simulink model "Likitha_Version_8_1"  (R2025b)
settings: Solver=VariableStepAuto  StartTime=0.0  StopTime=0.3  RelTol=1e-3
undefined symbols (not defined in the file): Ion, Lithium
libraries: spsBatteryLib x50, spsSeriesRLCBranchLib x15, spsCurrentMeasurementLib x10, spsVoltageMeasurementLib x10, spsIdealSwitchLib x9, spsMosfetLib x7, slpidlib x4, spsPWMGeneratorDCDCLib x2, spspowerguiLib x2, spsACVoltageSourceLib x1, eeHysteresisControl x1, spsDCMachineLib x1
(part 3 of 4)

== system Likitha_Version_8_1/Subsystem11/4 ==
  Battery1 : spsBatteryLib/Battery  BatType=Lithium-Ion  NomV=3.3  NomQ=2.7  SOC=98.5  Batt_Tr=30  PresetModel=on  MaxQ=2.7  MinV=2.475  FullV=3.8412  Dis_rate=1.1739  R=0.012222  Normal_OP=2.4417  expZone="[3.5653     0.13265]"
  Bus Selector : BusSelector  OutputSignals=SOC (%),Current (A),Voltage (V)
  Product : Product
  Scope : Scope  NumInputPorts=4
      settings: ActiveDisplayYMinimum=99.92989  ActiveDisplayYMaximum=100.00779
  + : PMIOPort  Side=Right
  - : PMIOPort  Port=2  Side=Right
  tag scope: cm_4=global, soc4=global, vm_4=global
  wires:
  Battery1/1 -> Bus Selector/1
  Bus Selector/1 -> [soc4], Scope/1  "<SOC (%)>"
  Product/1 -> Scope/4
  Bus Selector/2 -> [cm_4], Product/1, Scope/2  "<Current (A)>"
  Bus Selector/3 -> [vm_4], Scope/3, Product/2  "<Voltage (V)>"
  connections:
  +/RConn1 -- Battery1/LConn1
  -/RConn1 -- Battery1/LConn2

== system Likitha_Version_8_1/Subsystem11/40 ==
  Battery1 : spsBatteryLib/Battery  BatType=Lithium-Ion  NomV=3.21  NomQ=2.52  SOC=72  Batt_Tr=30  PresetModel=on  MaxQ=2.52  MinV=2.4075  FullV=3.7364  Dis_rate=1.0957  R=0.012738  Normal_OP=2.279  expZone="[3.468     0.12381]"
  Bus Selector : BusSelector  OutputSignals=SOC (%),Current (A),Voltage (V)
  Product : Product
  Scope : Scope  NumInputPorts=4
      settings: ActiveDisplayYMinimum=99.92989  ActiveDisplayYMaximum=100.00779
  + : PMIOPort  Side=Right
  - : PMIOPort  Port=2  Side=Right
  tag scope: cm_29=global, soc29=global, vm_29=global
  wires:
  Battery1/1 -> Bus Selector/1
  Bus Selector/1 -> [soc29], Scope/1  "<SOC (%)>"
  Product/1 -> Scope/4
  Bus Selector/2 -> [cm_29], Product/1, Scope/2  "<Current (A)>"
  Bus Selector/3 -> [vm_29], Scope/3, Product/2  "<Voltage (V)>"
  connections:
  +/RConn1 -- Battery1/LConn1
  -/RConn1 -- Battery1/LConn2

== system Likitha_Version_8_1/Subsystem11/41 ==
  Battery1 : spsBatteryLib/Battery  BatType=Lithium-Ion  NomV=3.15  NomQ=2.4  SOC=65  Batt_Tr=30  PresetModel=on  MaxQ=2.4  MinV=2.3625  FullV=3.6666  Dis_rate=1.0435  R=0.013125  Normal_OP=2.1704  expZone="[3.4032     0.11791]"
  Bus Selector : BusSelector  OutputSignals=SOC (%),Current (A),Voltage (V)
  Product : Product
  Scope : Scope  NumInputPorts=4
      settings: ActiveDisplayYMinimum=99.92989  ActiveDisplayYMaximum=100.00779
  Series RLC Branch : spsSeriesRLCBranchLib/Series RLC Branch  LConnTagsString=__new0  RConnTagsString=__new0  BranchType=R  Resistance=0.01  Inductance=1e-3  SetiL0=off  InitialCurrent=0  Capacitance=1e-6  Setx0=off  InitialVoltage=0  Measurements=None
  + : PMIOPort  Side=Right
  - : PMIOPort  Port=2  Side=Right
  tag scope: cm_41=global, soc41=global, vm_41=global
  wires:
  Battery1/1 -> Bus Selector/1
  Bus Selector/1 -> [soc41], Scope/1  "<SOC (%)>"
  Product/1 -> Scope/4
  Bus Selector/2 -> [cm_41], Product/1, Scope/2  "<Current (A)>"
  Bus Selector/3 -> [vm_41], Scope/3, Product/2  "<Voltage (V)>"
  connections:
  -/RConn1 -- Battery1/LConn2
  Series RLC Branch/LConn1 -- Battery1/LConn1
  Series RLC Branch/RConn1 -- +/RConn1

== system Likitha_Version_8_1/Subsystem11/42 ==
  Battery1 : spsBatteryLib/Battery  BatType=Lithium-Ion  NomV=3.105  NomQ=2.31  SOC=56  Batt_Tr=30  PresetModel=on  MaxQ=2.31  MinV=2.3287  FullV=3.6142  Dis_rate=1.0043  R=0.013442  Normal_OP=2.089  expZone="[3.3546     0.11349]"
  Bus Selector : BusSelector  OutputSignals=SOC (%),Current (A),Voltage (V)
  Product : Product
  Scope : Scope  NumInputPorts=4
      settings: ActiveDisplayYMinimum=-1  ActiveDisplayYMaximum=1
  + : PMIOPort  Side=Right
  - : PMIOPort  Port=2  Side=Right
  tag scope: cm_50=global, soc50=global, vm_50=global
  wires:
  Battery1/1 -> Bus Selector/1
  Bus Selector/1 -> [soc50], Scope/1  "<SOC (%)>"
  Product/1 -> Scope/4
  Bus Selector/2 -> [cm_50], Product/1, Scope/2  "<Current (A)>"
  Bus Selector/3 -> [vm_50], Scope/3, Product/2  "<Voltage (V)>"
  connections:
  +/RConn1 -- Battery1/LConn1
  -/RConn1 -- Battery1/LConn2

== system Likitha_Version_8_1/Subsystem11/43 ==
  Battery1 : spsBatteryLib/Battery  BatType=Lithium-Ion  NomV=3.145  NomQ=2.39  SOC=64  Batt_Tr=30  PresetModel=on  MaxQ=2.39  MinV=2.3588  FullV=3.6607  Dis_rate=1.0391  R=0.013159  Normal_OP=2.1614  expZone="[3.3978     0.11742]"
  Bus Selector : BusSelector  OutputSignals=SOC (%),Current (A),Voltage (V)
  Product : Product
  Scope : Scope  NumInputPorts=4
      settings: ActiveDisplayYMinimum=99.92989  ActiveDisplayYMaximum=100.00779
  + : PMIOPort  Side=Right
  - : PMIOPort  Port=2  Side=Right
  tag scope: cm_42=global, soc42=global, vm_42=global
  wires:
  Battery1/1 -> Bus Selector/1
  Bus Selector/1 -> [soc42], Scope/1  "<SOC (%)>"
  Product/1 -> Scope/4
  Bus Selector/2 -> [cm_42], Product/1, Scope/2  "<Current (A)>"
  Bus Selector/3 -> [vm_42], Scope/3, Product/2  "<Voltage (V)>"
  connections:
  +/RConn1 -- Battery1/LConn1
  -/RConn1 -- Battery1/LConn2

== system Likitha_Version_8_1/Subsystem11/44 ==
  Battery1 : spsBatteryLib/Battery  BatType=Lithium-Ion  NomV=3.14  NomQ=2.38  SOC=63  Batt_Tr=30  PresetModel=on  MaxQ=2.38  MinV=2.355  FullV=3.6549  Dis_rate=1.0348  R=0.013193  Normal_OP=2.1523  expZone="[3.3924     0.11693]"
  Bus Selector : BusSelector  OutputSignals=SOC (%),Current (A),Voltage (V)
  Product : Product
  Scope : Scope  NumInputPorts=4
      settings: ActiveDisplayYMinimum=99.92989  ActiveDisplayYMaximum=100.00779
  + : PMIOPort  Side=Right
  - : PMIOPort  Port=2  Side=Right
  tag scope: cm_43=global, soc43=global, vm_43=global
  wires:
  Battery1/1 -> Bus Selector/1
  Bus Selector/1 -> [soc43], Scope/1  "<SOC (%)>"
  Product/1 -> Scope/4
  Bus Selector/2 -> [cm_43], Product/1, Scope/2  "<Current (A)>"
  Bus Selector/3 -> [vm_43], Scope/3, Product/2  "<Voltage (V)>"
  connections:
  +/RConn1 -- Battery1/LConn1
  -/RConn1 -- Battery1/LConn2

== system Likitha_Version_8_1/Subsystem11/45 ==
  Battery1 : spsBatteryLib/Battery  BatType=Lithium-Ion  NomV=3.135  NomQ=2.37  SOC=62  Batt_Tr=30  PresetModel=on  MaxQ=2.37  MinV=2.3512  FullV=3.6491  Dis_rate=1.0304  R=0.013228  Normal_OP=2.1433  expZone="[3.387     0.11644]"
  Bus Selector : BusSelector  OutputSignals=SOC (%),Current (A),Voltage (V)
  Product : Product
  Scope : Scope  NumInputPorts=4
      settings: ActiveDisplayYMinimum=99.92989  ActiveDisplayYMaximum=100.00779
  + : PMIOPort  Side=Right
  - : PMIOPort  Port=2  Side=Right
  tag scope: cm_44=global, soc44=global, vm_44=global
  wires:
  Battery1/1 -> Bus Selector/1
  Bus Selector/1 -> [soc44], Scope/1  "<SOC (%)>"
  Product/1 -> Scope/4
  Bus Selector/2 -> [cm_44], Product/1, Scope/2  "<Current (A)>"
  Bus Selector/3 -> [vm_44], Scope/3, Product/2  "<Voltage (V)>"
  connections:
  +/RConn1 -- Battery1/LConn1
  -/RConn1 -- Battery1/LConn2

== system Likitha_Version_8_1/Subsystem11/46 ==
  Battery1 : spsBatteryLib/Battery  BatType=Lithium-Ion  NomV=3.13  NomQ=2.36  SOC=61  Batt_Tr=30  PresetModel=on  MaxQ=2.36  MinV=2.3475  FullV=3.6433  Dis_rate=1.0261  R=0.013263  Normal_OP=2.1343  expZone="[3.3816     0.11595]"
  Bus Selector : BusSelector  OutputSignals=SOC (%),Current (A),Voltage (V)
  Product : Product
  Scope : Scope  NumInputPorts=4
      settings: ActiveDisplayYMinimum=99.92989  ActiveDisplayYMaximum=100.00779
  + : PMIOPort  Side=Right
  - : PMIOPort  Port=2  Side=Right
  tag scope: cm_45=global, soc45=global, vm_45=global
  wires:
  Battery1/1 -> Bus Selector/1
  Bus Selector/1 -> [soc45], Scope/1  "<SOC (%)>"
  Product/1 -> Scope/4
  Bus Selector/2 -> [cm_45], Product/1, Scope/2  "<Current (A)>"
  Bus Selector/3 -> [vm_45], Scope/3, Product/2  "<Voltage (V)>"
  connections:
  +/RConn1 -- Battery1/LConn1
  -/RConn1 -- Battery1/LConn2

== system Likitha_Version_8_1/Subsystem11/47 ==
  Battery1 : spsBatteryLib/Battery  BatType=Lithium-Ion  NomV=3.125  NomQ=2.35  SOC=60  Batt_Tr=30  PresetModel=on  MaxQ=2.35  MinV=2.3438  FullV=3.6375  Dis_rate=1.0217  R=0.013298  Normal_OP=2.1252  expZone="[3.3762     0.11546]"
  Bus Selector : BusSelector  OutputSignals=SOC (%),Current (A),Voltage (V)
  Product : Product
  Scope : Scope  NumInputPorts=4
      settings: ActiveDisplayYMinimum=99.92989  ActiveDisplayYMaximum=100.00779
  + : PMIOPort  Side=Right
  - : PMIOPort  Port=2  Side=Right
  tag scope: cm_46=global, soc46=global, vm_46=global
  wires:
  Battery1/1 -> Bus Selector/1
  Bus Selector/1 -> [soc46], Scope/1  "<SOC (%)>"
  Product/1 -> Scope/4
  Bus Selector/2 -> [cm_46], Product/1, Scope/2  "<Current (A)>"
  Bus Selector/3 -> [vm_46], Scope/3, Product/2  "<Voltage (V)>"
  connections:
  +/RConn1 -- Battery1/LConn1
  -/RConn1 -- Battery1/LConn2

== system Likitha_Version_8_1/Subsystem11/48 ==
  Battery1 : spsBatteryLib/Battery  BatType=Lithium-Ion  NomV=3.12  NomQ=2.34  SOC=59  Batt_Tr=30  PresetModel=on  MaxQ=2.34  MinV=2.34  FullV=3.6316  Dis_rate=1.0174  R=0.013333  Normal_OP=2.1162  expZone="[3.3708     0.11497]"
  Bus Selector : BusSelector  OutputSignals=SOC (%),Current (A),Voltage (V)
  Product : Product
  Scope : Scope  NumInputPorts=4
      settings: ActiveDisplayYMinimum=99.92989  ActiveDisplayYMaximum=100.00779
  + : PMIOPort  Side=Right
  - : PMIOPort  Port=2  Side=Right
  tag scope: cm_47=global, soc47=global, vm_47=global
  wires:
  Battery1/1 -> Bus Selector/1
  Bus Selector/1 -> [soc47], Scope/1  "<SOC (%)>"
  Product/1 -> Scope/4
  Bus Selector/2 -> [cm_47], Product/1, Scope/2  "<Current (A)>"
  Bus Selector/3 -> [vm_47], Scope/3, Product/2  "<Voltage (V)>"
  connections:
  +/RConn1 -- Battery1/LConn1
  -/RConn1 -- Battery1/LConn2

== system Likitha_Version_8_1/Subsystem11/49 ==
  Battery1 : spsBatteryLib/Battery  BatType=Lithium-Ion  NomV=3.115  NomQ=2.33  SOC=58  Batt_Tr=30  PresetModel=on  MaxQ=2.33  MinV=2.3363  FullV=3.6258  Dis_rate=1.013  R=0.013369  Normal_OP=2.1071  expZone="[3.3654     0.11447]"
  Bus Selector : BusSelector  OutputSignals=SOC (%),Current (A),Voltage (V)
  Product : Product
  Scope : Scope  NumInputPorts=4
      settings: ActiveDisplayYMinimum=99.92989  ActiveDisplayYMaximum=100.00779
  + : PMIOPort  Side=Right
  - : PMIOPort  Port=2  Side=Right
  tag scope: cm_48=global, soc48=global, vm_48=global
  wires:
  Battery1/1 -> Bus Selector/1
  Bus Selector/1 -> [soc48], Scope/1  "<SOC (%)>"
  Product/1 -> Scope/4
  Bus Selector/2 -> [cm_48], Product/1, Scope/2  "<Current (A)>"
  Bus Selector/3 -> [vm_48], Scope/3, Product/2  "<Voltage (V)>"
  connections:
  +/RConn1 -- Battery1/LConn1
  -/RConn1 -- Battery1/LConn2

== system Likitha_Version_8_1/Subsystem11/5 ==
  Battery1 : spsBatteryLib/Battery  BatType=Lithium-Ion  NomV=3.3  NomQ=2.7  SOC=98  Batt_Tr=30  PresetModel=on  MaxQ=2.7  MinV=2.475  FullV=3.8412  Dis_rate=1.1739  R=0.012222  Normal_OP=2.4417  expZone="[3.5653     0.13265]"
  Bus Selector : BusSelector  OutputSignals=SOC (%),Current (A),Voltage (V)
  Product : Product
  Scope : Scope  NumInputPorts=4
      settings: ActiveDisplayYMinimum=99.92989  ActiveDisplayYMaximum=100.00779
  + : PMIOPort  Side=Right
  - : PMIOPort  Port=2  Side=Right
  tag scope: cm_5=global, soc5=global, vm_5=global
  wires:
  Battery1/1 -> Bus Selector/1
  Bus Selector/1 -> [soc5], Scope/1  "<SOC (%)>"
  Bus Selector/2 -> Product/1, Scope/2  "<Current (A)>"
  Product/1 -> Scope/4
  Bus Selector/3 -> [vm_5], [cm_5], Scope/3, Product/2  "<Voltage (V)>"
  connections:
  +/RConn1 -- Battery1/LConn1
  -/RConn1 -- Battery1/LConn2

== system Likitha_Version_8_1/Subsystem11/50 ==
  Battery1 : spsBatteryLib/Battery  BatType=Lithium-Ion  NomV=3.11  NomQ=2.32  SOC=57  Batt_Tr=30  PresetModel=on  MaxQ=2.32  MinV=2.3325  FullV=3.62  Dis_rate=1.0087  R=0.013405  Normal_OP=2.0981  expZone="[3.36     0.11398]"
  Bus Selector : BusSelector  OutputSignals=SOC (%),Current (A),Voltage (V)
  Product : Product
  Scope : Scope  NumInputPorts=4
      settings: ActiveDisplayYMinimum=99.92989  ActiveDisplayYMaximum=100.00779
  + : PMIOPort  Side=Right
  - : PMIOPort  Port=2  Side=Right
  tag scope: cm_49=global, soc49=global, vm_49=global
  wires:
  Battery1/1 -> Bus Selector/1
  Bus Selector/1 -> [soc49], Scope/1  "<SOC (%)>"
  Product/1 -> Scope/4
  Bus Selector/2 -> [cm_49], Product/1, Scope/2  "<Current (A)>"
  Bus Selector/3 -> [vm_49], Scope/3, Product/2  "<Voltage (V)>"
  connections:
  +/RConn1 -- Battery1/LConn1
  -/RConn1 -- Battery1/LConn2

== system Likitha_Version_8_1/Subsystem11/6 ==
  Battery1 : spsBatteryLib/Battery  BatType=Lithium-Ion  NomV=3.3  NomQ=2.7  SOC=97.5  Batt_Tr=30  PresetModel=on  MaxQ=2.7  MinV=2.475  FullV=3.8412  Dis_rate=1.1739  R=0.012222  Normal_OP=2.4417  expZone="[3.5653     0.13265]"
  Bus Selector : BusSelector  OutputSignals=SOC (%),Current (A),Voltage (V)
  Product : Product
  Scope : Scope  NumInputPorts=4
      settings: ActiveDisplayYMinimum=99.92989  ActiveDisplayYMaximum=100.00779
  + : PMIOPort  Side=Right
  - : PMIOPort  Port=2  Side=Right
  tag scope: cm_6=global, soc6=global, vm_6=global
  wires:
  Battery1/1 -> Bus Selector/1
  Bus Selector/1 -> [soc6], Scope/1  "<SOC (%)>"
  Product/1 -> Scope/4
  Bus Selector/2 -> [cm_6], Product/1, Scope/2  "<Current (A)>"
  Bus Selector/3 -> [vm_6], Scope/3, Product/2  "<Voltage (V)>"
  connections:
  +/RConn1 -- Battery1/LConn1
  -/RConn1 -- Battery1/LConn2

== system Likitha_Version_8_1/Subsystem11/7 ==
  Battery1 : spsBatteryLib/Battery  BatType=Lithium-Ion  NomV=3.3  NomQ=2.7  SOC=97  Batt_Tr=30  PresetModel=on  MaxQ=2.7  MinV=2.475  FullV=3.8412  Dis_rate=1.1739  R=0.012222  Normal_OP=2.4417  expZone="[3.5653     0.13265]"
  Bus Selector : BusSelector  OutputSignals=SOC (%),Current (A),Voltage (V)
  Product : Product
  Scope : Scope  NumInputPorts=4
      settings: ActiveDisplayYMinimum=99.92989  ActiveDisplayYMaximum=100.00779
  + : PMIOPort  Side=Right
  - : PMIOPort  Port=2  Side=Right
  tag scope: cm_7=global, soc7=global, vm_7=global
  wires:
  Battery1/1 -> Bus Selector/1
  Bus Selector/1 -> [soc7], Scope/1  "<SOC (%)>"
  Product/1 -> Scope/4
  Bus Selector/2 -> [cm_7], Product/1, Scope/2  "<Current (A)>"
  Bus Selector/3 -> [vm_7], Scope/3, Product/2  "<Voltage (V)>"
  connections:
  +/RConn1 -- Battery1/LConn1
  -/RConn1 -- Battery1/LConn2

== system Likitha_Version_8_1/Subsystem11/8 ==
  Battery1 : spsBatteryLib/Battery  BatType=Lithium-Ion  NomV=3.3  NomQ=2.7  SOC=96.5  Batt_Tr=30  PresetModel=on  MaxQ=2.7  MinV=2.475  FullV=3.8412  Dis_rate=1.1739  R=0.012222  Normal_OP=2.4417  expZone="[3.5653     0.13265]"
  Bus Selector : BusSelector  OutputSignals=SOC (%),Current (A),Voltage (V)
  Product : Product
  Scope : Scope  NumInputPorts=4
      settings: ActiveDisplayYMinimum=99.92989  ActiveDisplayYMaximum=100.00779
  + : PMIOPort  Side=Right
  - : PMIOPort  Port=2  Side=Right
  tag scope: cm_8=global, soc8=global, vm_8=global
  wires:
  Battery1/1 -> Bus Selector/1
  Bus Selector/1 -> [soc8], Scope/1  "<SOC (%)>"
  Product/1 -> Scope/4
  Bus Selector/2 -> [cm_8], Product/1, Scope/2  "<Current (A)>"
  Bus Selector/3 -> Scope/3, [vm_8], Product/2  "<Voltage (V)>"
  connections:
  +/RConn1 -- Battery1/LConn1
  -/RConn1 -- Battery1/LConn2

== system Likitha_Version_8_1/Subsystem11/9 ==
  Battery1 : spsBatteryLib/Battery  BatType=Lithium-Ion  NomV=3.3  NomQ=2.7  SOC=96  Batt_Tr=30  PresetModel=on  MaxQ=2.7  MinV=2.475  FullV=3.8412  Dis_rate=1.1739  R=0.012222  Normal_OP=2.4417  expZone="[3.5653     0.13265]"
  Bus Selector : BusSelector  OutputSignals=SOC (%),Current (A),Voltage (V)
  Product : Product
  Scope : Scope  NumInputPorts=4
      settings: ActiveDisplayYMinimum=99.92989  ActiveDisplayYMaximum=100.00779
  + : PMIOPort  Side=Right
  - : PMIOPort  Port=2  Side=Right
  tag scope: cm_9=global, soc9=global, vm_9=global
  wires:
  Battery1/1 -> Bus Selector/1
  Bus Selector/1 -> [soc9], Scope/1  "<SOC (%)>"
  Product/1 -> Scope/4
  Bus Selector/2 -> [cm_9], Product/1, Scope/2  "<Current (A)>"
  Bus Selector/3 -> [vm_9], Scope/3, Product/2  "<Voltage (V)>"
  connections:
  +/RConn1 -- Battery1/LConn1
  -/RConn1 -- Battery1/LConn2

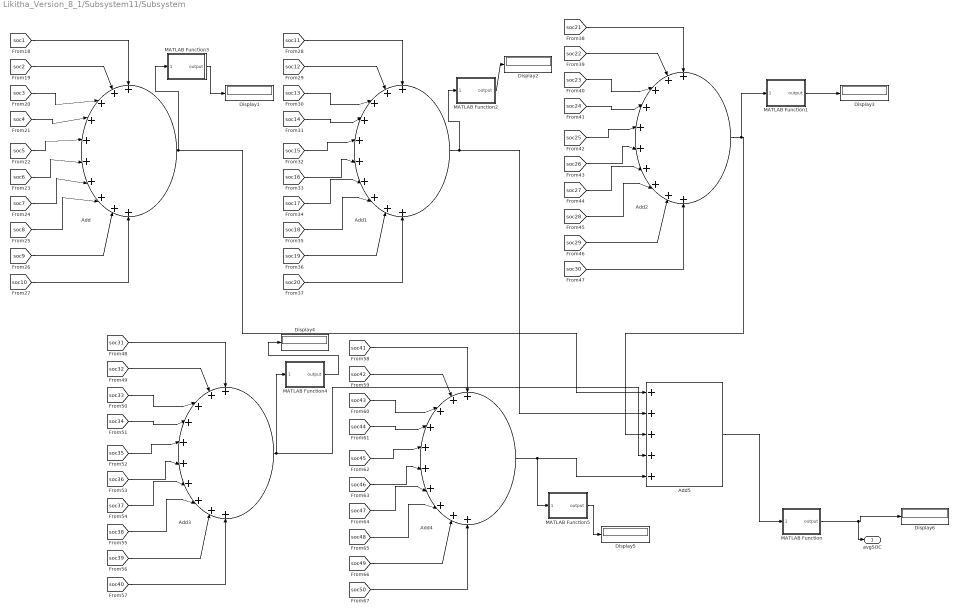
== system Likitha_Version_8_1/Subsystem11/Subsystem ==
  Add{,1..4} (5 alike) : Sum  Inputs=++++++++++
  Add5 : Sum  Inputs=+++++
  Display{1..6} (6 alike) : Display
  MATLAB Function : MATLAB Function  TreatAsAtomicUnit=on
  MATLAB Function1 : MATLAB Function  TreatAsAtomicUnit=on
  MATLAB Function2 : MATLAB Function  TreatAsAtomicUnit=on
  MATLAB Function3 : MATLAB Function  TreatAsAtomicUnit=on
  MATLAB Function4 : MATLAB Function  TreatAsAtomicUnit=on
  MATLAB Function5 : MATLAB Function  TreatAsAtomicUnit=on
  avgSOC : Outport
  wires:
  [soc16] -> Add1/6
  [soc31] -> Add3/1
  [soc42] -> Add4/2
  [soc6] -> Add/6
  Add3/1 -> MATLAB Function4/1(inputValue), Add5/4
  [soc33] -> Add3/3
  [soc12] -> Add1/2
  [soc50] -> Add4/10
  [soc1] -> Add/1
  [soc13] -> Add1/3
  [soc39] -> Add3/9
  Add2/1 -> MATLAB Function1/1(inputValue), Add5/3
  [soc28] -> Add2/8
  [soc3] -> Add/3
  [soc17] -> Add1/7
  [soc36] -> Add3/6
  [soc2] -> Add/2
  [soc45] -> Add4/5
  [soc49] -> Add4/9
  [soc27] -> Add2/7
  [soc48] -> Add4/8
  [soc15] -> Add1/5
  [soc20] -> Add1/10
  [soc43] -> Add4/3
  [soc26] -> Add2/6
  Add1/1 -> MATLAB Function2/1(inputValue), Add5/2
  [soc41] -> Add4/1
  [soc46] -> Add4/6
  [soc14] -> Add1/4
  [soc24] -> Add2/4
  [soc22] -> Add2/2
  [soc44] -> Add4/4
  [soc47] -> Add4/7
  [soc38] -> Add3/8
  [soc21] -> Add2/1
  [soc18] -> Add1/8
  [soc7] -> Add/7
  [soc19] -> Add1/9
  [soc9] -> Add/9
  [soc40] -> Add3/10
  [soc4] -> Add/4
  [soc11] -> Add1/1
  [soc35] -> Add3/5
  [soc8] -> Add/8
  Add/1 -> Add5/1, MATLAB Function3/1(inputValue)
  [soc5] -> Add/5
  [soc37] -> Add3/7
  [soc29] -> Add2/9
  Add4/1 -> MATLAB Function5/1(inputValue), Add5/5
  [soc34] -> Add3/4
  [soc32] -> Add3/2
  [soc10] -> Add/10
  [soc25] -> Add2/5
  [soc30] -> Add2/10
  [soc23] -> Add2/3
  Add5/1 -> MATLAB Function/1(inputValue)
  MATLAB Function/1(output) -> avgSOC/1, Display6/1
  MATLAB Function1/1(output) -> Display3/1
  MATLAB Function2/1(output) -> Display2/1
  MATLAB Function3/1(output) -> Display1/1
  MATLAB Function4/1(output) -> Display4/1
  MATLAB Function5/1(output) -> Display5/1

== system Likitha_Version_8_1/AC to DC/Subsystem1/Subsystem ==
  Iref : Inport
  Clock : Clock
  Constant : Constant  Value=2*pi/3
  Gain : Gain  Gain=2*pi*50
  Gain2 : Gain  Gain=2*pi*50
  Gain3 : Gain  Gain=2*pi*50
  Mux : Mux  Inputs=3
  Product : Product
  Sin : Trigonometry
  Sin1 : Trigonometry
  Sin2 : Trigonometry
  Subtract : Sum  Inputs=+-
  Subtract1 : Sum
  Out1 : Outport
  wires:
  Mux/1 -> Product/1
  Gain/1 -> Sin/1
  Sin2/1 -> Mux/3
  Clock/1 -> Gain3/1, Gain2/1, Gain/1
  Sin/1 -> Mux/1
  Constant/1 -> Subtract1/2, Subtract/2
  Subtract/1 -> Sin1/1
  Sin1/1 -> Mux/2
  Gain2/1 -> Subtract/1
  Gain3/1 -> Subtract1/1
  Subtract1/1 -> Sin2/1
  Product/1 -> Out1/1
  Iref/1 -> Product/2

== matlab function Likitha_Version_8_1/Subsystem11/MATLAB Function ==
  settings: updateMethod=DISCRETE
  data: V1 input; S1 output; V2 input; V3 input; V4 input; V5 input; S2 output; S3 output; S4 output; S5 output
function [S1,S2,S3,S4,S5] = battery_pack_switch_logic(V1,V2,V3,V4,V5)
% Outputs: 1 = ON, 0 = OFF

%% Parameters
V_over = 35;      % Over-voltage threshold
V_under = 30;     % Under-voltage threshold
V_tol = 0.5;      % Voltage balancing tolerance

V = [V1 V2 V3 V4 V5];

%% Persistent switch states (memory)
persistent S
if isempty(S)
    S = ones(1,5);   % All ON initially
end

%% Average voltage of active packs
V_active = V(S == 1);
if isempty(V_active)
    V_avg = mean(V);   % fallback
else
    V_avg = mean(V_active);
end

%% Control logic
for i = 1:5

    % Protection: Over / Under Voltage
    if V(i) > V_over || V(i) < V_under
        S(i) = 0;   % Force OFF
    end

    % Re-enable logic (balancing condition)
    if S(i) == 0
        if abs(V(i) - V_avg) <= V_tol
            S(i) = 1;   % Turn ON again
        end
    end

end

%% Outputs
S1 = S(1);
S2 = S(2);
S3 = S(3);
S4 = S(4);
S5 = S(5);

end

== matlab function Likitha_Version_8_1/Subsystem2/MATLAB Function1 ==
  settings: updateMethod=DISCRETE
  data: SOC input double size=1; windowData output double size=[100 22]; SOH input double size=1; SOP input double size=1; DOD input double size=1; ROH input double size=1; RUL input double size=1; CycleCount input double size=1; V_avg input double size=1; I_avg input double size=1; P_avg input double size=1; stress_idx input double size=1; aging_rate_frac input double size=1; energy_kWh input double size=1; degrad_idx input double size=1; T_idx input double size=1; health_idx input double size=1; I_peak input double size=1; V_min input double size=1; T_max input double size=1; Ah_charge_total input double size=1; Ah_discharge_total input double size=1; overtime_sec input double size=1; timestamp input double size=1; windowLabels output double size=[1 2]; dataValid output double size=1
function [windowData, windowLabels, dataValid] = PreTrainingData_Fixed(...
    SOC, SOH, SOP, DOD, ROH, RUL, CycleCount, ...
    V_avg, I_avg, P_avg, stress_idx, aging_rate_frac, energy_kWh, ...
    degrad_idx, T_idx, health_idx, I_peak, V_min, T_max, ...
    Ah_charge_total, Ah_discharge_total, overtime_sec, ...
    timestamp)

% Internal constants
windowSize = 100;   % number of samples per window
stepSize   = 0.1;   % time interval (s) between new windows

persistent buffer timeBuffer bufferIdx counter lastOutputTime
persistent firstRun

if isempty(firstRun)
    buffer = zeros(windowSize, 22);
    timeBuffer = zeros(windowSize, 1);
    bufferIdx = 1;
    counter = 0;
    lastOutputTime = -inf;
    firstRun = false;
end

% Current feature vector (1×22)
currentFeatures = [SOC, SOH, SOP, DOD, ROH, RUL, CycleCount, ...
                   V_avg, I_avg, P_avg, stress_idx, aging_rate_frac, energy_kWh, ...
                   degrad_idx, T_idx, health_idx, I_peak, V_min, T_max, ...
                   Ah_charge_total, Ah_discharge_total, overtime_sec];

% Store in circular buffer
buffer(bufferIdx, :) = currentFeatures;
timeBuffer(bufferIdx) = timestamp;
bufferIdx = mod(bufferIdx, windowSize) + 1;
counter = counter + 1;

% Default outputs (fixed size)
windowData = zeros(windowSize, 22);
windowLabels = [0, 0];
dataValid = 0;

% Check if we have a full window and enough time has passed
if counter >= windowSize && (timestamp - lastOutputTime) >= stepSize
    % Create index order for chronological order
    if bufferIdx > 1
        idxOrder = [bufferIdx:windowSize, 1:bufferIdx-1];
    else
        idxOrder = 1:windowSize;
    end
    % Fill windowData row by row (ensures fixed size)
    for i = 1:windowSize
        windowData(i, :) = buffer(idxOrder(i), :);
    end
    windowLabels = windowData(end, 1:2);
    dataValid = 1;
    lastOutputTime = timestamp;
end

end

== matlab function Likitha_Version_8_1/Subsystem2/MATLAB Function2 ==
  data: windowData input double size=[100 22]; SOC_pred output double size=1; windowLabels input double size=[1 2]; dataValid input double size=1; algorithmChoice input double size=1; SOH_pred output double size=1; RUL_pred output double size=1; confidence output double size=[1 2]; algoCode output double size=1; metrics output double size=[1 4]
function [SOC_pred, SOH_pred, RUL_pred, confidence, algoCode, metrics] = ...
    AI_ML_Estimator(windowData, windowLabels, dataValid, algorithmChoice)

% AI/ML/DL Estimator – fixed‑size, code‑generation compatible, no tic/toc
%
% Inputs:
%   windowData      : [100x22] matrix – most recent window of parameters
%   windowLabels    : [1x2] vector – [SOC, SOH] of the last sample in window
%   dataValid       : scalar – 1 when a new window is ready
%   algorithmChoice : scalar – 1=Linear, 2=Neural, 3=LSTM
%
% Outputs (all fixed size):
%   SOC_pred, SOH_pred, RUL_pred : scalars
%   confidence                    : [1x2] vector [conf_SOC, conf_SOH]
%   algoCode                      : scalar (0=None, 1=Linear, 2=Neural, 3=LSTM)
%   metrics                       : [1x4] vector [RMSE_SOC, RMSE_SOH, MAE_SOC, MAE_SOH]

% -------------------------------------------------------------------------
% Internal constants (must match Block 8)
windowSize = 100;
retrainInterval = 10;   % retrain every 'retrainInterval' new windows
% -------------------------------------------------------------------------

persistent X_buffer Y_buffer bufferIdx nSamples
persistent theta_SOC theta_SOH
persistent windowCount trainedAlgo

% Initialize all persistent variables
if isempty(X_buffer)
    X_buffer = zeros(windowSize, 22);
    Y_buffer = zeros(windowSize, 2);
    bufferIdx = 1;
    nSamples = 0;
    theta_SOC = zeros(22, 1);
    theta_SOH = zeros(22, 1);
    windowCount = 0;
    trainedAlgo = 0;
end

% Initialize outputs (to avoid "undefined on some paths")
SOC_pred = 0;
SOH_pred = 0;
RUL_pred = 0;
confidence = [0.5, 0.5];
algoCode = 0;
metrics = zeros(1, 4);   % ensures metrics is always defined

% If a new valid window arrives, store its last sample as a training point
if dataValid
    X_last = windowData(end, :);      % 1x22
    Y_last = windowLabels;             % 1x2

    % Store in circular buffer
    X_buffer(bufferIdx, :) = X_last;
    Y_buffer(bufferIdx, :) = Y_last;
    bufferIdx = mod(bufferIdx, windowSize) + 1;
    nSamples = min(nSamples + 1, windowSize);

    windowCount = windowCount + 1;
end

% Retrain when enough windows and sufficient samples
if dataValid && nSamples >= 30 && windowCount >= retrainInterval
    X_train = X_buffer(1:nSamples, :);
    Y_train = Y_buffer(1:nSamples, :);
    X_aug = [ones(nSamples, 1), X_train];   % add bias

    switch algorithmChoice
        case 1  % Linear Regression
            theta_SOC = (X_aug' * X_aug) \ (X_aug' * Y_train(:,1));
            theta_SOH = (X_aug' * X_aug) \ (X_aug' * Y_train(:,2));
            trainedAlgo = 1;

        case 2  % Neural Net (placeholder – use linear)
            theta_SOC = (X_aug' * X_aug) \ (X_aug' * Y_train(:,1));
            theta_SOH = (X_aug' * X_aug) \ (X_aug' * Y_train(:,2));
            trainedAlgo = 2;   % still linear for now

        case 3  % LSTM placeholder
            theta_SOC = (X_aug' * X_aug) \ (X_aug' * Y_train(:,1));
            theta_SOH = (X_aug' * X_aug) \ (X_aug' * Y_train(:,2));
            trainedAlgo = 3;
    end

    % Compute metrics
    Y_pred_SOC = X_aug * theta_SOC;
    Y_pred_SOH = X_aug * theta_SOH;
    rmse_soc = sqrt(mean((Y_train(:,1) - Y_pred_SOC).^2));
    rmse_soh = sqrt(mean((Y_train(:,2) - Y_pred_SOH).^2));
    mae_soc  = mean(abs(Y_train(:,1) - Y_pred_SOC));
    mae_soh  = mean(abs(Y_train(:,2) - Y_pred_SOH));
    metrics = [rmse_soc, rmse_soh, mae_soc, mae_soh];

    windowCount = 0;   % reset counter
end

% Make prediction using the most recent sample
X_pred = windowData(end, :);          % 1x22
X_pred_aug = [1, X_pred];             % add bias

if trainedAlgo >= 1
    SOC_pred = X_pred_aug * theta_SOC;
    SOH_pred = X_pred_aug * theta_SOH;
    confidence = [0.9, 0.9];
    algoCode = trainedAlgo;
else
    % No model yet – use the labels of the current window
    SOC_pred = windowLabels(1);
    SOH_pred = windowLabels(2);
    confidence = [0.7, 0.7];
    algoCode = 0;
    metrics = zeros(1,4);
end

% Clamp
SOC_pred = max(0, min(100, SOC_pred));
SOH_pred = max(0, min(100, SOH_pred));

% Estimate RUL from SOH
if SOH_pred > 80
    RUL_pred = (SOH_pred - 80) / 0.1;
else
    RUL_pred = 0;
end
RUL_pred = max(0, RUL_pred);

end

== matlab function Likitha_Version_8_1/Subsystem1/MATLAB Function ==
  settings: updateMethod=DISCRETE  sampleTime=0.1
  data: V_meas input; SOC_est output; I_meas input; P_meas input; SOC_ext input; T_meas input; dt input; Vp1_est output; Vp2_est output; R0_est output; Cap_est output; OCV_est output; Vfilt output
function [SOC_est, Vp1_est, Vp2_est, R0_est, Cap_est, OCV_est, Vfilt] = AEKF_Battery(V_meas, I_meas, P_meas, SOC_ext, T_meas, dt)
% AEKF_Battery - Adaptive Extended Kalman Filter for Li-ion battery state estimation
% 
% Inputs:
%   V_meas  : Measured terminal voltage (V)
%   I_meas  : Measured current (A)  [positive = discharge, negative = charge]
%   P_meas  : Measured power (W)     (optional, not used in filter)
%   SOC_ext : External SOC measurement (%) e.g., from Coulomb counter
%   T_meas  : Measured temperature (°C)
%   dt      : Simulation time step (s)
%
% Outputs:
%   SOC_est : Estimated State of Charge (%)
%   Vp1_est : Estimated polarization voltage across R1-C1 (V)
%   Vp2_est : Estimated polarization voltage across R2-C2 (V)
%   R0_est  : Estimated internal resistance (Ohm)
%   Cap_est : Estimated capacity (Ah)
%   OCV_est : Estimated open circuit voltage (V)
%   Vfilt   : Filtered voltage (V) using updated states

% -------------------------------------------------------------------------
% Persistent variables (retained between calls)
% -------------------------------------------------------------------------
persistent x P Q R R_SOC
persistent R0 R1 C1 R2 C2         % Model parameters (may depend on SOC/T)
persistent nominal_capacity        % Ah
persistent first_run

% -------------------------------------------------------------------------
% Initialization (tune these values to match your cell)
% -------------------------------------------------------------------------
if isempty(first_run)
    first_run = false;
    nominal_capacity = 50;   % Nominal capacity (Ah)
    
    % Initial state [SOC(%); Vp1(V); Vp2(V); bias(V); invCap(1/Ah)]
    x = [100; 0; 0; 0; 1/nominal_capacity];
    
    % Initial covariance
    P = diag([1, 0.1, 0.1, 0.01, 1e-6]);
    
    % Process noise covariance (will be adapted)
    Q = diag([0.01, 0.001, 0.001, 1e-6, 1e-8]);
    
    % Measurement noise variances
    R     = 0.1;   % Voltage measurement noise (V^2)
    R_SOC = 1.0;   % External SOC measurement noise (%^2) – tune based on sensor
    
    % Fixed model parameters (you may replace with SOC/T lookup)
    R0 = 0.05;   % Ohm
    R1 = 0.02;   % Ohm
    C1 = 2000;   % Farad
    C2 = 0.03;   % Ohm? Wait, fix: R2 = 0.03 Ohm, C2 = 5000 F
    R2 = 0.03;   % Ohm
    C2 = 5000;   % Farad
end

% -------------------------------------------------------------------------
% Time constant checks (avoid division by zero)
% -------------------------------------------------------------------------
tau1 = max(R1*C1, 1e-6);
tau2 = max(R2*C2, 1e-6);

% -------------------------------------------------------------------------
% 1. Prediction step (a priori estimate)
% -------------------------------------------------------------------------
% Extract states
SOC = x(1);
Vp1 = x(2);
Vp2 = x(3);
bias = x(4);
invCap = x(5);
Cap = 1 / max(invCap, 1e-6);   % Capacity in Ah

% State transition
alpha1 = exp(-dt / tau1);
alpha2 = exp(-dt / tau2);

x_pred = [SOC - (I_meas * dt) / (3600 * Cap);
          alpha1 * Vp1 + (1 - alpha1) * R1 * I_meas;
          alpha2 * Vp2 + (1 - alpha2) * R2 * I_meas;
          bias;
          invCap];

% Jacobian
F = [1, 0, 0, 0,  (I_meas * dt) / (3600 * Cap^2);
     0, alpha1, 0, 0, 0;
     0, 0, alpha2, 0, 0;
     0, 0, 0, 1, 0;
     0, 0, 0, 0, 1];

P_pred = F * P * F' + Q;

% -------------------------------------------------------------------------
% 2. OCV model (as function of SOC)
% -------------------------------------------------------------------------
% Replace with lookup table for higher accuracy
OCV = polyval([-1.5e-6, 2e-4, -0.01, 0.3, 0.1, 3.0], SOC);
dOCV_dSOC = polyval([-7.5e-6, 8e-4, -0.03, 0.6, 0.1], SOC);

% -------------------------------------------------------------------------
% 3. Measurement update (stacked voltage and external SOC)
% -------------------------------------------------------------------------
% Predicted measurements
V_pred = OCV - I_meas * R0 - Vp1 - Vp2 + bias;
SOC_pred = SOC;   % direct state

% Stacked measurement vector
z = [V_meas; SOC_ext];
z_pred = [V_pred; SOC_pred];

% Measurement Jacobian H = [dV/dx; dSOC/dx]
H = [dOCV_dSOC, -1, -1, 1, 0;   % first row: voltage
     1,         0,  0,  0, 0];   % second row: SOC (direct)

% Measurement noise covariance matrix
R_mat = [R,    0;
         0, R_SOC];

% Innovation
y = z - z_pred;

% Innovation covariance
S = H * P_pred * H' + R_mat;

% Kalman gain
K = P_pred * H' / S;

% State update
x_upd = x_pred + K * y;

% Covariance update
P_upd = (eye(5) - K * H) * P_pred;

% -------------------------------------------------------------------------
% 4. Adaptive noise covariance estimation (optional for voltage)
% -------------------------------------------------------------------------
persistent r_sum r_count
if isempty(r_sum)
    r_sum = 0;
    r_count = 0;
end
r_sum = r_sum + y(1)^2;   % voltage innovation
r_count = r_count + 1;
if r_count > 100
    R_est = r_sum / r_count;
    R = 0.95 * R + 0.05 * R_est;
    r_sum = 0;
    r_count = 0;
end

% -------------------------------------------------------------------------
% 5. Apply constraints
% -------------------------------------------------------------------------
x_upd(1) = max(0, min(100, x_upd(1)));   % SOC bounds
x_upd(5) = max(1/(2*nominal_capacity), min(1/(0.5*nominal_capacity), x_upd(5)));

x = x_upd;
P = P_upd;

% -------------------------------------------------------------------------
% Output assignments
% -------------------------------------------------------------------------
SOC_est = x(1);
Vp1_est = x(2);
Vp2_est = x(3);
bias_est = x(4);
Cap_est = 1 / x(5);
R0_est = R0;
OCV_est = OCV;
Vfilt = OCV_est - I_meas * R0 - Vp1_est - Vp2_est + bias_est;

% Note: Power input P_meas is not used in this filter but can be added
% to thermal model or used for redundancy in future versions.

end

== matlab function Likitha_Version_8_1/Subsystem2/MATLAB Function ==
  settings: updateMethod=DISCRETE  sampleTime=0.1
  data: SOC output; SOH output; SOP output; SOC_in input; DOD output; ROH output; Vp1 input double size=1; Vp2 input; R0_in input; RUL output; CycleCount output; V_avg output; Cap_in input; I_meas input; V_meas input; T_meas input; dt input; I_avg output; P_avg output; stress_idx output double size=1; aging_rate_frac output; energy_kWh output; degrad_idx output; T_idx output; health_idx output; I_peak output; V_min output; T_max output; Ah_charge_total output; Ah_discharge_total output; overtime_sec output
function [SOC, SOH, SOP, DOD, ROH, RUL, CycleCount, ...
          V_avg, I_avg, P_avg, stress_idx, aging_rate_frac, energy_kWh, ...
          degrad_idx, T_idx, health_idx, I_peak, V_min, T_max, ...
          Ah_charge_total, Ah_discharge_total, overtime_sec] = ...
          ParameterEstimator(...
          SOC_in, Vp1, Vp2, R0_in, Cap_in, I_meas, V_meas, T_meas, dt)
% ParameterEstimator - Computes all battery health and performance parameters
% 
% Inputs:
%   SOC_in   : Estimated SOC from filter (%)
%   Vp1, Vp2 : Polarization voltages (V)
%   R0_in    : Internal resistance (Ohm)
%   Cap_in   : Estimated capacity (Ah)
%   I_meas   : Measured current (A)
%   V_meas   : Measured voltage (V)
%   T_meas   : Measured temperature (°C)
%   dt       : Time step (s)
%
% Outputs (22 total):
%   SOC        : State of Charge (%) – passed through
%   SOH        : State of Health (%) – based on capacity fade
%   SOP        : State of Power (W) – max discharge power
%   DOD        : Depth of Discharge (%) = 100 - SOC
%   ROH        : Internal resistance (Ohm) – filtered version
%   RUL        : Remaining Useful Life (cycles)
%   CycleCount : Number of equivalent full cycles
%   V_avg      : Average voltage (V)
%   I_avg      : Average current (A)
%   P_avg      : Average power (W)
%   stress_idx : Stress index (0-1)
%   aging_rate_frac : Aging rate (fraction per cycle)
%   energy_kWh : Cumulative energy throughput (kWh)
%   degrad_idx : Degradation index (1 - SOH/100)
%   T_idx      : Temperature index (0-1, optimum 25°C)
%   health_idx : Overall health index (0-1)
%   I_peak     : Peak current (A, with decay)
%   V_min      : Minimum voltage (V, with recovery)
%   T_max      : Maximum temperature (°C, with decay)
%   Ah_charge_total  : Total charge Ampere-hours (Ah)
%   Ah_discharge_total: Total discharge Ampere-hours (Ah)
%   overtime_sec     : Cumulative time above 45°C (s)

% -------------------------------------------------------------------------
% Persistent variables for historical data
% -------------------------------------------------------------------------
persistent nominal_capacity cycleCount Ah_throughput lastSOC
persistent V_avg_pers I_avg_pers P_avg_pers E_throughput I_peak_pers V_min_pers T_max_pers
persistent Ah_charge Ah_discharge overtemp_time
persistent first_run

% -------------------------------------------------------------------------
% Initialization
% -------------------------------------------------------------------------
if isempty(first_run)
    nominal_capacity = 50;        % Nominal capacity at BOL (Ah)
    cycleCount = 0;
    Ah_throughput = 0;
    lastSOC = 100;
    
    V_avg_pers = V_meas;
    I_avg_pers = I_meas;
    P_avg_pers = V_meas * I_meas;
    E_throughput = 0;
    I_peak_pers = abs(I_meas);
    V_min_pers = V_meas;
    T_max_pers = T_meas;
    Ah_charge = 0;
    Ah_discharge = 0;
    overtemp_time = 0;
    
    first_run = true;
end

% -------------------------------------------------------------------------
% Basic passed-through parameters
% -------------------------------------------------------------------------
SOC = SOC_in;                       % %
DOD = 100 - SOC;                    % %
ROH = R0_in;                         % Ohm (could apply low-pass filter)
SOH = (Cap_in / nominal_capacity) * 100;   % %
SOH = max(0, min(100, SOH));

% -------------------------------------------------------------------------
% Cycle counting (full cycle when SOC crosses 20% -> 80%)
% -------------------------------------------------------------------------
if lastSOC <= 20 && SOC >= 80
    cycleCount = cycleCount + 1;
end
lastSOC = SOC;
CycleCount = cycleCount;

% -------------------------------------------------------------------------
% Update Ah throughput and energy throughput
% -------------------------------------------------------------------------
dAh = abs(I_meas) * dt / 3600;          % Ampere-hours
Ah_throughput = Ah_throughput + dAh;

dEnergy = abs(V_meas * I_meas) * dt / 3600 / 1000;   % kWh
E_throughput = E_throughput + dEnergy;

% Separate charge/discharge Ah
if I_meas < 0   % charging
    Ah_charge = Ah_charge + abs(I_meas) * dt / 3600;
elseif I_meas > 0
    Ah_discharge = Ah_discharge + I_meas * dt / 3600;
end

% -------------------------------------------------------------------------
% State of Power (SOP) estimation
% -------------------------------------------------------------------------
% Use OCV from SOC (simplified linear model – replace with lookup if available)
OCV = 0.04 * SOC + 3.0;   % V
Vmin = 2.7;   % Minimum allowed voltage
I_max_dis = (OCV - Vmin) / (ROH + 1e-6);   % A
SOP = I_max_dis * Vmin;   % W (max discharge power)

% -------------------------------------------------------------------------
% Remaining Useful Life (RUL) based on aging rate
% -------------------------------------------------------------------------
% Compute aging rate per cycle from capacity fade
if cycleCount > 0
    aging_rate_per_cycle = (100 - SOH) / cycleCount;   % % loss per cycle
else
    aging_rate_per_cycle = 0.01;   % default 0.01% per cycle
end
cycles_to_80 = (SOH - 80) / aging_rate_per_cycle;
RUL = max(0, cycles_to_80);

% -------------------------------------------------------------------------
% 15 Additional health parameters (exponential moving averages, peaks, etc.)
% -------------------------------------------------------------------------
alpha = 0.01;   % smoothing factor for averages (~100 samples time constant)

% 1. Average voltage
V_avg_pers = (1 - alpha) * V_avg_pers + alpha * V_meas;
V_avg = V_avg_pers;

% 2. Average current
I_avg_pers = (1 - alpha) * I_avg_pers + alpha * I_meas;
I_avg = I_avg_pers;

% 3. Average power
P_avg_pers = (1 - alpha) * P_avg_pers + alpha * (V_meas * I_meas);
P_avg = P_avg_pers;

% 4. Stress index (function of C-rate and temperature)
C_rate = abs(I_meas) / Cap_in;   % Current in C-rate
stress_idx = min(1, (C_rate / 2) * (T_meas / 50));

% 5. Aging rate (as fraction per cycle)
aging_rate_frac = aging_rate_per_cycle / 100;

% 6. Energy throughput (already computed in kWh)
energy_kWh = E_throughput;

% 7. Degradation index
degrad_idx = 1 - SOH/100;

% 8. Temperature index (normalized 0-1, optimum 25°C)
T_idx = max(0, min(1, 1 - abs(T_meas - 25)/50));

% 9. Overall health index (weighted combination)
health_idx = 0.5*(SOH/100) + 0.3*(1-stress_idx) + 0.2*T_idx;

% 10. Peak current (with slow decay)
I_peak_pers = max(abs(I_meas), 0.999 * I_peak_pers);
I_peak = I_peak_pers;

% 11. Minimum voltage (with slow recovery)
V_min_pers = min(V_meas, V_min_pers + 0.001);
V_min = V_min_pers;

% 12. Maximum temperature (with slow decay)
T_max_pers = max(T_meas, T_max_pers - 0.01);
T_max = T_max_pers;

% 13. Charge throughput (Ah)
Ah_charge_total = Ah_charge;

% 14. Discharge throughput (Ah)
Ah_discharge_total = Ah_discharge;

% 15. Time at over-temperature (cumulative seconds above 45°C)
if T_meas > 45
    overtemp_time = overtemp_time + dt;
end
overtime_sec = overtemp_time;

% Ensure all outputs are real
SOC = real(SOC);
SOH = real(SOH);
SOP = real(SOP);
DOD = real(DOD);
ROH = real(ROH);
RUL = real(RUL);
CycleCount = real(CycleCount);
V_avg = real(V_avg);
I_avg = real(I_avg);
P_avg = real(P_avg);
stress_idx = real(stress_idx);
aging_rate_frac = real(aging_rate_frac);
energy_kWh = real(energy_kWh);
degrad_idx = real(degrad_idx);
T_idx = real(T_idx);
health_idx = real(health_idx);
I_peak = real(I_peak);
V_min = real(V_min);
T_max = real(T_max);
Ah_charge_total = real(Ah_charge_total);
Ah_discharge_total = real(Ah_discharge_total);
overtime_sec = real(overtime_sec);

end

== matlab function Likitha_Version_8_1/Subsystem11/Subsystem/MATLAB Function1 ==
  data: inputValue input; output output
function output = divideByFifty(inputValue)
% This function divides the input decimal value by 10

output = inputValue / 10;

end

== matlab function Likitha_Version_8_1/Subsystem11/Subsystem/MATLAB Function2 ==
  data: inputValue input; output output
function output = divideByFifty(inputValue)
% This function divides the input decimal value by 10

output = inputValue / 10;

end

== matlab function Likitha_Version_8_1/Subsystem11/Subsystem/MATLAB Function3 ==
  data: inputValue input; output output
function output = divideByFifty(inputValue)
% This function divides the input decimal value by 10

output = inputValue / 10;

end

== matlab function Likitha_Version_8_1/Subsystem11/Subsystem/MATLAB Function4 ==
  data: inputValue input; output output
function output = divideByFifty(inputValue)
% This function divides the input decimal value by 10

output = inputValue / 10;

end

== matlab function Likitha_Version_8_1/Subsystem11/Subsystem/MATLAB Function5 ==
  data: inputValue input; output output
function output = divideByFifty(inputValue)
% This function divides the input decimal value by 10

output = inputValue / 10;

end

== matlab function Likitha_Version_8_1/Subsystem2/MATLAB Function3 ==
  data: SOC input; SOC_pred output; SOH input; SOP input; DOD input; ROH input; RUL input; CycleCount input; V_avg input; I_avg input; P_avg input; stress_idx input; aging_rate_frac input; energy_kWh input; degrad_idx input; T_idx input; health_idx input; I_peak input; V_min input; T_max input; Ah_charge_total input; Ah_discharge_total input; overtime_sec input; timestamp input; enableTraining input; algorithmChoice input; SOH_pred output; RUL_pred output; conf_SOC output; conf_SOH output; modelTypeCode output
function [SOC_pred, SOH_pred, RUL_pred, conf_SOC, conf_SOH, modelTypeCode] = ...
    AI_ML_Predictor_CodeGen(...
    SOC, SOH, SOP, DOD, ROH, RUL, CycleCount, ...
    V_avg, I_avg, P_avg, stress_idx, aging_rate_frac, energy_kWh, ...
    degrad_idx, T_idx, health_idx, I_peak, V_min, T_max, ...
    Ah_charge_total, Ah_discharge_total, overtime_sec, ...
    timestamp, enableTraining, algorithmChoice)

% Code-generation compatible online linear regression
% Inputs: 22 parameters + timestamp + enableTraining + algorithmChoice
% Outputs: SOC_pred, SOH_pred, RUL_pred, conf_SOC, conf_SOH, modelTypeCode

% Persistent variables (fixed-size)
persistent X_buffer Y_buffer bufferIdx nSamples
persistent theta_SOC theta_SOH
persistent lastTrainTime

% Initialize fixed-size buffers (max 200 samples)
if isempty(X_buffer)
    X_buffer = zeros(200, 22);   % fixed size: 200 x 22
    Y_buffer = zeros(200, 2);
    bufferIdx = 1;
    nSamples = 0;
    theta_SOC = zeros(22, 1);
    theta_SOH = zeros(22, 1);
    lastTrainTime = 0.0;
end

% Current feature vector (row)
X_curr = [SOC, SOH, SOP, DOD, ROH, RUL, CycleCount, ...
          V_avg, I_avg, P_avg, stress_idx, aging_rate_frac, energy_kWh, ...
          degrad_idx, T_idx, health_idx, I_peak, V_min, T_max, ...
          Ah_charge_total, Ah_discharge_total, overtime_sec];

% Store in buffer if training enabled
if enableTraining && (timestamp > 0)
    X_buffer(bufferIdx, :) = X_curr;
    Y_buffer(bufferIdx, :) = [SOC, SOH];
    bufferIdx = mod(bufferIdx, 200) + 1;
    if nSamples < 200
        nSamples = nSamples + 1;
    end
end

% Retrain every 5 seconds if enough samples
retrainInterval = 5.0; % seconds
if enableTraining && (nSamples >= 30) && ((timestamp - lastTrainTime) >= retrainInterval)
    % Use all stored samples
    X_train = X_buffer(1:nSamples, :);
    Y_train = Y_buffer(1:nSamples, :);
    
    % Add bias term (intercept) – create augmented matrix
    X_aug = [ones(nSamples, 1), X_train];   % size nSamples x 23
    
    % Ordinary Least Squares: theta = (X'*X)\X'*Y
    % Using pseudo-inverse for numerical stability (supported in codegen)
    theta_SOC = (X_aug' * X_aug) \ (X_aug' * Y_train(:, 1));
    theta_SOH = (X_aug' * X_aug) \ (X_aug' * Y_train(:, 2));
    
    lastTrainTime = timestamp;
end

% Make prediction
if any(theta_SOC ~= 0)   % model exists
    X_pred = [1, X_curr];   % row with bias
    SOC_pred = X_pred * theta_SOC;
    SOH_pred = X_pred * theta_SOH;
    conf_SOC = 0.9;
    conf_SOH = 0.9;
    modelTypeCode = 1;   % 1 = linear regression
else
    % Fallback: moving average of last 10 samples
    if nSamples >= 10
        startIdx = max(1, nSamples-9);
        SOC_pred = mean(Y_buffer(startIdx:nSamples, 1));
        SOH_pred = mean(Y_buffer(startIdx:nSamples, 2));
    else
        SOC_pred = SOC;
        SOH_pred = SOH;
    end
    conf_SOC = 0.7;
    conf_SOH = 0.7;
    modelTypeCode = 0;   % 0 = moving average
end

% Clamp predictions
SOC_pred = max(0.0, min(100.0, SOC_pred));
SOH_pred = max(0.0, min(100.0, SOH_pred));

% Estimate RUL from SOH
if SOH_pred > 80.0
    RUL_pred = (SOH_pred - 80.0) / 0.1;   % assume 0.1% loss per cycle
else
    RUL_pred = 0.0;
end
RUL_pred = max(0.0, RUL_pred);

end

== matlab function Likitha_Version_8_1/Subsystem3/MATLAB Function ==
  settings: updateMethod=DISCRETE
  data: t input; V output; I output; P output; SOC output; T output
function [V, I, P, SOC, T] = HardwareEmulator(t)
% HardwareEmulator - Generates synthetic battery data for testing
% 
% Input:
%   t : current simulation time (s) from a Clock block
%
% Outputs:
%   V   : pack voltage (V)
%   I   : pack current (A) - positive for discharge
%   P   : pack power (W)
%   SOC : state of charge (%)
%   T   : temperature (°C) - constant 25

% -------------------------------------------------------------------------
% Internal parameters (adjust to match your battery pack)
capacity = 50;          % nominal capacity (Ah)
I_nom = 30;             % discharge current (A)
% Linear voltage model: V = a * SOC + b   (at SOC in %)
a = 0.2;                % V/% (voltage change per % SOC)
b = 140;                % V at 0% SOC
T_nom = 25;             % constant temperature (°C)
% -------------------------------------------------------------------------

persistent lastTime lastSOC

% Initialize on first call
if isempty(lastTime)
    lastTime = t;
    lastSOC = 100;      % start fully charged
end

% Time step
dt = t - lastTime;
if dt < 0
    dt = 0;   % protect against negative time (should not happen)
end

% Update SOC using Coulomb counting
% dSOC (%) = (I * dt) / (capacity * 3600) * 100
dSOC = (I_nom * dt) / (capacity * 3600) * 100;
lastSOC = lastSOC - dSOC;   % discharge reduces SOC

% Keep SOC within [0, 100]
lastSOC = max(0, min(100, lastSOC));

% Compute outputs
SOC = lastSOC;
I = I_nom;
V = a * SOC + b;
P = V * I;
T = T_nom;

% Update last time for next step
lastTime = t;

end
